simulink model "test_pltl"  (R2014a)
settings: Solver=FixedStepDiscrete  StartTime=0.0  StopTime=inf  RelTol=1e-3
libraries: patterns_library x6
settings Model: Creator=lgwagner  LastModifiedBy=lgwagner

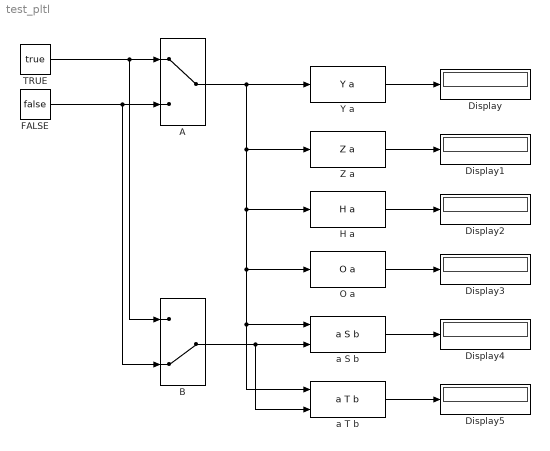
== system test_pltl ==
  A : ManualSwitch
  B : ManualSwitch  CurrentSetting=0
  Display{,1..5} (6 alike) : Display
  FALSE : Constant  Value=false
  H a : patterns_library/H a
  O a : patterns_library/O a
  "TRUE " : Constant  Value=true
  Y a : patterns_library/Y a
  Z a : patterns_library/Z a
  a S b : patterns_library/a S b
  a T b : patterns_library/a T b
  wires:
  "TRUE "/1 -> B/1, A/1
  FALSE/1 -> B/2, A/2
  A/1 -> Y a/1, Z a/1, H a/1, O a/1, a T b/1, a S b/1
  B/1 -> a T b/2, a S b/2
  Y a/1 -> Display/1
  Z a/1 -> Display1/1
  H a/1 -> Display2/1
  O a/1 -> Display3/1
  a S b/1 -> Display4/1
  a T b/1 -> Display5/1
